simulink model "Cor1_Ex1"  (R2020b)
settings: Solver=FixedStepAuto  StartTime=0.0  StopTime=4  FixedStep=0.001  RelTol=1e-3
values from neighbouring files (symbols this model uses):
  K = [K11 K12 K13 ... (first row only)    [Cor1_deflmivar_cvx.m]
  P = [P11  P12  P13 ... (first row only)    [Cor1_deflmivar_cvx.m]
  x0 = [1; 2]    [Cor1.m]
undefined symbols (not defined in the file or in its folder): avar, bvar
libraries: simulink x1
settings Model: Creator=kyungsoo  LastModifiedBy=kyungsoo

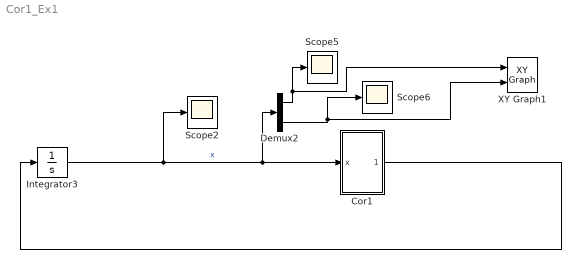
== system Cor1_Ex1 ==
  Cor1 : Subsystem
  Demux2 : Demux  Outputs=2
  Integrator3 : Integrator  InitialCondition=x0
  Scope2 : Scope
  Scope5 : Scope
  Scope6 : Scope
  XY Graph1 : simulink/Sinks/XY Graph  xmin=-10  xmax=10  ymin=-10  ymax=10  st=-1
  wires:
  Integrator3/1 -> Scope2/1, Demux2/1, Cor1/1(x)  "x"
  Demux2/2 -> XY Graph1/2, Scope6/1
  Cor1/1(x_dot) -> Integrator3/1
  Demux2/1 -> Scope5/1, XY Graph1/1

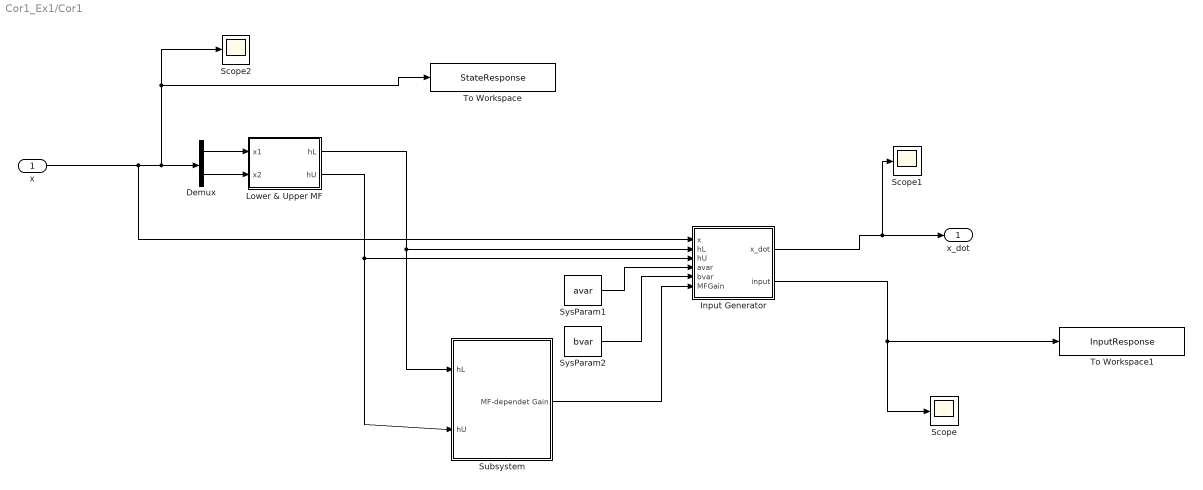
== system Cor1_Ex1/Cor1 ==
  x : Inport
  Demux : Demux  Outputs=2
  Input Generator : MATLAB Function  TreatAsAtomicUnit=on
  Lower & Upper MF : MATLAB Function  TreatAsAtomicUnit=on
  Scope : Scope
  Scope1 : Scope
  Scope2 : Scope
  Subsystem : Subsystem
  SysParam1 : Constant  Value=avar  VectorParams1D=off
  SysParam2 : Constant  Value=bvar  VectorParams1D=off
  To Workspace : ToWorkspace  VariableName=StateResponse  SaveFormat=Timeseries  SampleTime=-1
  To Workspace1 : ToWorkspace  VariableName=InputResponse  SaveFormat=Timeseries  SampleTime=-1
  x_dot : Outport
  wires:
  Demux/1 -> Lower & Upper MF/1(x1)
  Demux/2 -> Lower & Upper MF/2(x2)
  x/1 -> Input Generator/1(x), To Workspace/1, Scope2/1, Demux/1
  Lower & Upper MF/1(hL) -> Input Generator/2(hL), Subsystem/1(hL)
  Lower & Upper MF/2(hU) -> Subsystem/2(hU), Input Generator/3(hU)
  SysParam1/1 -> Input Generator/4(avar)
  SysParam2/1 -> Input Generator/5(bvar)
  Subsystem/1(MF-dependet Gain) -> Input Generator/6(MFGain)
  Input Generator/1(x_dot) -> Scope1/1, x_dot/1
  Input Generator/2(input) -> Scope/1, To Workspace1/1

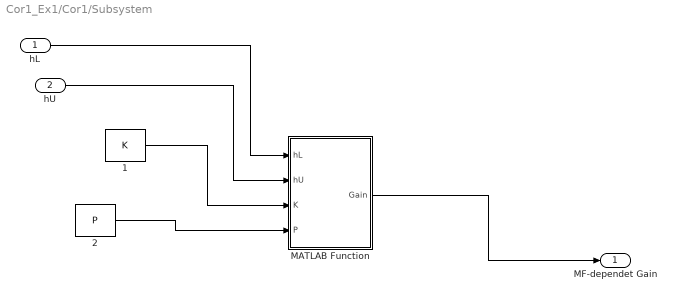
== system Cor1_Ex1/Cor1/Subsystem ==
  hL : Inport
  hU : Inport  Port=2
  1 : Constant  Value=K  VectorParams1D=off
  2 : Constant  Value=P  VectorParams1D=off
  MATLAB Function : MATLAB Function  TreatAsAtomicUnit=on
  MF-dependet Gain : Outport
  wires:
  2/1 -> MATLAB Function/4(P)
  hL/1 -> MATLAB Function/1(hL)
  MATLAB Function/1(Gain) -> MF-dependet Gain/1
  1/1 -> MATLAB Function/3(K)
  hU/1 -> MATLAB Function/2(hU)

== matlab function Cor1_Ex1/Cor1/Input Generator ==
  data: x_dot output; x input; hL input; input output; hU input; avar input; bvar input; MFGain input
function [x_dot, input]= fcn(x, hL, hU, avar ,bvar, MFGain)

h = (hL + hU)/2;
I_nx = eye(2);  I_nu = eye(1);

A1 = [2.78 -5.63; 0.01 0.33];
A2 = [0.2  -3.22; 0.35 0.12];
B1 = [2;    -1];
B2 = [8;     0];
A3 = [-avar   -6.63; 0.45 0.15];
B3 = [-bvar+6; -1];

Ah = [A1 A2 A3]*kron(h,I_nx);
Bh = [B1 B2 B3]*kron(h,I_nu);

x_dot = (Ah + Bh*MFGain)*x;

input = MFGain*x;

== matlab function Cor1_Ex1/Cor1/Lower & Upper MF ==
  data: x1 input; hL output; hU output; x2 input
function [hL, hU]= fcn(x1, x2)
if x1>10
    x1 = 10;
end
if x1<-10
    x1 = -10;
end

LMF_1 = 0.95 - (0.925./(1+exp(-((x1+4.5)/8))));   
UMF_1 = 0.95 - (0.925./(1+exp(-((x1+3.5)/8))));    

LMF_3 = 0.025 + (0.925./(1+exp(-((x1-4.5)/8))));
UMF_3 = 0.025 + (0.925./(1+exp(-((x1-3.5)/8))));

LMF_2 = 1 - (UMF_1 + UMF_3);
UMF_2 = 1 - (LMF_1 + LMF_3);


hL = [LMF_1; LMF_2; LMF_3];
hU = [UMF_1; UMF_2; UMF_3];

== matlab function Cor1_Ex1/Cor1/Subsystem/MATLAB Function ==
  data: hL input; hU input; K input; Gain output; P input
function Gain = fcn(hL, hU, K, P)

Inx = eye(2);
Inu = eye(1);
 
Outer_nu = [Inu; kron(hL,Inu); kron(hU,Inu)];
Outer_nx = [Inx; kron(hL,Inx); kron(hU,Inx)];

Gain = (Outer_nu'*K*Outer_nx)*inv(Outer_nx'*(P)*Outer_nx);
